simulink model "IEEE34_PQload"  (R2021b)
settings: Solver=ode4  StartTime=0.0  StopTime=5  FixedStep=50e-6  RelTol=1e-3
PreLoadFcn:
  | pGain = 0.05; % Gain of random perturbation (pu)
  | pGainAP = 0.01; % Gain of sinusoidal active power variation (pu)
  | pGainRP = 0.01; % Gain of sinusoidal reactive power variation (pu)
  | pFreqAP = 0.03; % Frequency of sinusoidal active power variation (Hz)
  | pFreqRP = 0.03; % Frequency of sinusoidal reactive power variation (Hz)
  | 
  | init_IEEE34nodetestfeeder;
InitFcn:
  | pGain = 0.05; % Gain of random perturbation (pu)
  | pGainAP = 0.01; % Gain of sinusoidal active power variation (pu)
  | pGainRP = 0.01; % Gain of sinusoidal reactive power variation (pu)
  | pFreqAP = 0.03; % Frequency of sinusoidal active power variation (Hz)
  | pFreqRP = 0.03; % Frequency of sinusoidal reactive power variation (Hz)
  | 
  | init_IEEE34nodetestfeeder;
values from neighbouring files (symbols this model uses):
  fNom = f    (= 60)    [init_IEEE34nodetestfeeder.m]
  loadcoeff = 1.0    (= 1)    [init_IEEE34nodetestfeeder.m]
  Pbase = 500e3    (= 500000)    [init_IEEE34nodetestfeeder.m]
  Ts = 50e-6    (= 5e-05)    [init_IEEE34nodetestfeeder.m]
  vNomMV = VsubL    (= 24900)    [init_IEEE34nodetestfeeder.m]
  VsubL = 24.9e3    (= 24900)    [init_IEEE34nodetestfeeder.m]
undefined symbols (not defined in the file or in its folder): find_system
libraries: spsSeriesRLCBranchLib x330, spsGroundLib x242, LoadLib x88, spsThreePhaseVIMeasurementLib x37, spsMutualInductanceLib x24, spsVoltageMeasurementLib x18, spsCurrentMeasurementLib x12, spsOnDelayLib x12, spsRMSLib x8, spsLinearTransformerLib x6, spsControlledCurrentSourceLib x6, spsControlledVoltageSourceLib x6
(part 2 of 8)

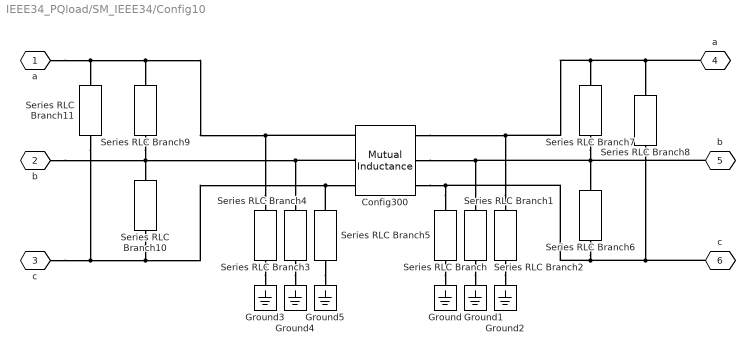
== system IEEE34_PQload/SM_IEEE34/Config10 ==
  Config300 : spsMutualInductanceLib/Mutual Inductance  LConnTagsString=a|b|c  RConnTagsString=A|B|C  TypeOfMutual=Generalized mutual inductance  NumberOfWindings=3  SelfImpedance1=[1.1 1.1e-03]  SelfImpedance2=[ 1.1 1.1e-03]  ThreeWindings=on  SelfImpedance3=[ 1.1 1.1e-03]  MutualImpedance=[1.0 1.0e-03]  InductanceMatrix=[1.3343 0.5779 0.5015 ; 0.5779 1.3569 0.4591; 0.5015 0.4591 1.3471] / (2*fNom*pi) * length/1.6  ResistanceMatrix="[1.3368 0.2101  0.2130 ;  0.2101 1.3238  0.2066;  0.2130 0.2066 1.3294] * length/1.6"  Measurements=None
      settings: SourceProductBaseCode=PS
  Ground{,1..5} (6 alike) : spsGroundLib/Ground  LConnTagsString=a
  Series RLC Branch : spsSeriesRLCBranchLib/Series RLC Branch  LConnTagsString=__new0  RConnTagsString=__new0  BranchType=C  Resistance=1  Inductance=1e-3  SetiL0=off  InitialCurrent=0  Capacitance=1.0417e-8 * length/1.6 / 2  Setx0=off  InitialVoltage=0  Measurements=None
  Series RLC Branch1 : spsSeriesRLCBranchLib/Series RLC Branch  LConnTagsString=__new0  RConnTagsString=__new0  BranchType=C  Resistance=1  Inductance=1e-3  SetiL0=off  InitialCurrent=0  Capacitance=9.3755e-9 * length/1.6 / 2  Setx0=off  InitialVoltage=0  Measurements=None
  Series RLC Branch10 : spsSeriesRLCBranchLib/Series RLC Branch  LConnTagsString=__new0  RConnTagsString=__new0  BranchType=C  Resistance=1  Inductance=1e-3  SetiL0=off  InitialCurrent=0  Capacitance=1.9773e-9 * length/1.6 / 2  Setx0=off  InitialVoltage=0  Measurements=None
  Series RLC Branch11 : spsSeriesRLCBranchLib/Series RLC Branch  LConnTagsString=__new0  RConnTagsString=__new0  BranchType=C  Resistance=1  Inductance=1e-3  SetiL0=off  InitialCurrent=0  Capacitance=3.1650e-9 * length/1.6 / 2  Setx0=off  InitialVoltage=0  Measurements=None
  Series RLC Branch2 : spsSeriesRLCBranchLib/Series RLC Branch  LConnTagsString=__new0  RConnTagsString=__new0  BranchType=C  Resistance=1  Inductance=1e-3  SetiL0=off  InitialCurrent=0  Capacitance=8.9426e-9 * length/1.6 / 2  Setx0=off  InitialVoltage=0  Measurements=None
  Series RLC Branch3 : spsSeriesRLCBranchLib/Series RLC Branch  LConnTagsString=__new0  RConnTagsString=__new0  BranchType=C  Resistance=1  Inductance=1e-3  SetiL0=off  InitialCurrent=0  Capacitance=8.9426e-9 * length/1.6 / 2  Setx0=off  InitialVoltage=0  Measurements=None
  Series RLC Branch4 : spsSeriesRLCBranchLib/Series RLC Branch  LConnTagsString=__new0  RConnTagsString=__new0  BranchType=C  Resistance=1  Inductance=1e-3  SetiL0=off  InitialCurrent=0  Capacitance=9.3755e-9 * length/1.6 / 2  Setx0=off  InitialVoltage=0  Measurements=None
  Series RLC Branch5 : spsSeriesRLCBranchLib/Series RLC Branch  LConnTagsString=__new0  RConnTagsString=__new0  BranchType=C  Resistance=1  Inductance=1e-3  SetiL0=off  InitialCurrent=0  Capacitance=1.0417e-8 * length/1.6 / 2  Setx0=off  InitialVoltage=0  Measurements=None
  Series RLC Branch6 : spsSeriesRLCBranchLib/Series RLC Branch  LConnTagsString=__new0  RConnTagsString=__new0  BranchType=C  Resistance=1  Inductance=1e-3  SetiL0=off  InitialCurrent=0  Capacitance=1.9773e-9 * length/1.6 / 2  Setx0=off  InitialVoltage=0  Measurements=None
  Series RLC Branch7 : spsSeriesRLCBranchLib/Series RLC Branch  LConnTagsString=__new0  RConnTagsString=__new0  BranchType=C  Resistance=1  Inductance=1e-3  SetiL0=off  InitialCurrent=0  Capacitance=4.8743e-9 * length/1.6 / 2  Setx0=off  InitialVoltage=0  Measurements=None
  Series RLC Branch8 : spsSeriesRLCBranchLib/Series RLC Branch  LConnTagsString=__new0  RConnTagsString=__new0  BranchType=C  Resistance=1  Inductance=1e-3  SetiL0=off  InitialCurrent=0  Capacitance=3.1650e-9 * length/1.6 / 2  Setx0=off  InitialVoltage=0  Measurements=None
  Series RLC Branch9 : spsSeriesRLCBranchLib/Series RLC Branch  LConnTagsString=__new0  RConnTagsString=__new0  BranchType=C  Resistance=1  Inductance=1e-3  SetiL0=off  InitialCurrent=0  Capacitance=4.8743e-9 * length/1.6 / 2  Setx0=off  InitialVoltage=0  Measurements=None
  a : PMIOPort  Tag=PMCPort  Side=Left
  b : PMIOPort  Tag=PMCPort  Port=2  Side=Left
  c : PMIOPort  Tag=PMCPort  Port=3  Side=Left
  "a " : PMIOPort  Tag=PMCPort  Port=4  Side=Right
  "b " : PMIOPort  Tag=PMCPort  Port=5  Side=Right
  "c " : PMIOPort  Tag=PMCPort  Port=6  Side=Right
  connections:
  Series RLC Branch3/LConn1 -- Config300/LConn1 -- Series RLC Branch9/LConn1 -- a/RConn1 -- Series RLC Branch11/LConn1
  b/RConn1 -- Series RLC Branch4/LConn1 -- Config300/LConn2 -- Series RLC Branch9/RConn1 -- Series RLC Branch10/LConn1
  Series RLC Branch5/LConn1 -- Config300/LConn3 -- Series RLC Branch10/RConn1 -- c/RConn1 -- Series RLC Branch11/RConn1
  Series RLC Branch2/LConn1 -- Config300/RConn1 -- Series RLC Branch7/LConn1 -- "a "/RConn1 -- Series RLC Branch8/LConn1
  "b "/RConn1 -- Series RLC Branch1/LConn1 -- Config300/RConn2 -- Series RLC Branch6/LConn1 -- Series RLC Branch7/RConn1
  Series RLC Branch/LConn1 -- Config300/RConn3 -- Series RLC Branch6/RConn1 -- "c "/RConn1 -- Series RLC Branch8/RConn1
  Series RLC Branch/RConn1 -- Ground/LConn1
  Series RLC Branch1/RConn1 -- Ground1/LConn1
  Series RLC Branch2/RConn1 -- Ground2/LConn1
  Series RLC Branch3/RConn1 -- Ground3/LConn1
  Series RLC Branch4/RConn1 -- Ground4/LConn1
  Series RLC Branch5/RConn1 -- Ground5/LConn1

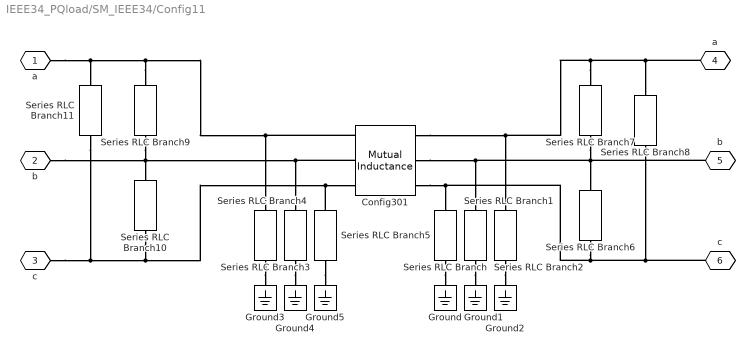
== system IEEE34_PQload/SM_IEEE34/Config11 ==
  Config301 : spsMutualInductanceLib/Mutual Inductance  LConnTagsString=a|b|c  RConnTagsString=A|B|C  TypeOfMutual=Generalized mutual inductance  NumberOfWindings=3  SelfImpedance1=[1.1 1.1e-03]  SelfImpedance2=[ 1.1 1.1e-03]  ThreeWindings=on  SelfImpedance3=[ 1.1 1.1e-03]  MutualImpedance=[1.0 1.0e-03]  InductanceMatrix=[1.4115 0.6442 0.5691 ; 0.6442 1.4281 0.5238; 0.5691 0.5238 1.4209] / (2*fNom*pi) * length/1.6  ResistanceMatrix="[1.9300 0.2327 0.2359 ; 0.2327 1.9157  0.2288;  0.2359 0.2288 1.9219] * length/1.6"  Measurements=None
      settings: SourceProductBaseCode=PS
  Ground{,1..5} (6 alike) : spsGroundLib/Ground  LConnTagsString=a
  Series RLC Branch : spsSeriesRLCBranchLib/Series RLC Branch  LConnTagsString=__new0  RConnTagsString=__new0  BranchType=C  Resistance=1  Inductance=1e-3  SetiL0=off  InitialCurrent=0  Capacitance=1.0123e-8 * length/1.6 / 2  Setx0=off  InitialVoltage=0  Measurements=None
  Series RLC Branch1 : spsSeriesRLCBranchLib/Series RLC Branch  LConnTagsString=__new0  RConnTagsString=__new0  BranchType=C  Resistance=1  Inductance=1e-3  SetiL0=off  InitialCurrent=0  Capacitance=9.1482e-9 * length/1.6 / 2  Setx0=off  InitialVoltage=0  Measurements=None
  Series RLC Branch10 : spsSeriesRLCBranchLib/Series RLC Branch  LConnTagsString=__new0  RConnTagsString=__new0  BranchType=C  Resistance=1  Inductance=1e-3  SetiL0=off  InitialCurrent=0  Capacitance=1.8943e-9 * length/1.6 / 2  Setx0=off  InitialVoltage=0  Measurements=None
  Series RLC Branch11 : spsSeriesRLCBranchLib/Series RLC Branch  LConnTagsString=__new0  RConnTagsString=__new0  BranchType=C  Resistance=1  Inductance=1e-3  SetiL0=off  InitialCurrent=0  Capacitance=2.9927e-9 * length/1.6 / 2  Setx0=off  InitialVoltage=0  Measurements=None
  Series RLC Branch2 : spsSeriesRLCBranchLib/Series RLC Branch  LConnTagsString=__new0  RConnTagsString=__new0  BranchType=C  Resistance=1  Inductance=1e-3  SetiL0=off  InitialCurrent=0  Capacitance=8.7347e-9 * length/1.6 / 2  Setx0=off  InitialVoltage=0  Measurements=None
  Series RLC Branch3 : spsSeriesRLCBranchLib/Series RLC Branch  LConnTagsString=__new0  RConnTagsString=__new0  BranchType=C  Resistance=1  Inductance=1e-3  SetiL0=off  InitialCurrent=0  Capacitance=8.7347e-9 * length/1.6 / 2  Setx0=off  InitialVoltage=0  Measurements=None
  Series RLC Branch4 : spsSeriesRLCBranchLib/Series RLC Branch  LConnTagsString=__new0  RConnTagsString=__new0  BranchType=C  Resistance=1  Inductance=1e-3  SetiL0=off  InitialCurrent=0  Capacitance=9.1482e-9 * length/1.6 / 2  Setx0=off  InitialVoltage=0  Measurements=None
  Series RLC Branch5 : spsSeriesRLCBranchLib/Series RLC Branch  LConnTagsString=__new0  RConnTagsString=__new0  BranchType=C  Resistance=1  Inductance=1e-3  SetiL0=off  InitialCurrent=0  Capacitance=1.0123e-8 * length/1.6 / 2  Setx0=off  InitialVoltage=0  Measurements=None
  Series RLC Branch6 : spsSeriesRLCBranchLib/Series RLC Branch  LConnTagsString=__new0  RConnTagsString=__new0  BranchType=C  Resistance=1  Inductance=1e-3  SetiL0=off  InitialCurrent=0  Capacitance=1.8943e-9 * length/1.6 / 2  Setx0=off  InitialVoltage=0  Measurements=None
  Series RLC Branch7 : spsSeriesRLCBranchLib/Series RLC Branch  LConnTagsString=__new0  RConnTagsString=__new0  BranchType=C  Resistance=1  Inductance=1e-3  SetiL0=off  InitialCurrent=0  Capacitance=4.5722e-9 * length/1.6 / 2  Setx0=off  InitialVoltage=0  Measurements=None
  Series RLC Branch8 : spsSeriesRLCBranchLib/Series RLC Branch  LConnTagsString=__new0  RConnTagsString=__new0  BranchType=C  Resistance=1  Inductance=1e-3  SetiL0=off  InitialCurrent=0  Capacitance=2.9927e-9 * length/1.6 / 2  Setx0=off  InitialVoltage=0  Measurements=None
  Series RLC Branch9 : spsSeriesRLCBranchLib/Series RLC Branch  LConnTagsString=__new0  RConnTagsString=__new0  BranchType=C  Resistance=1  Inductance=1e-3  SetiL0=off  InitialCurrent=0  Capacitance=4.5722e-9 * length/1.6 / 2  Setx0=off  InitialVoltage=0  Measurements=None
  a : PMIOPort  Tag=PMCPort  Side=Left
  b : PMIOPort  Tag=PMCPort  Port=2  Side=Left
  c : PMIOPort  Tag=PMCPort  Port=3  Side=Left
  "a " : PMIOPort  Tag=PMCPort  Port=4  Side=Right
  "b " : PMIOPort  Tag=PMCPort  Port=5  Side=Right
  "c " : PMIOPort  Tag=PMCPort  Port=6  Side=Right
  connections:
  Series RLC Branch9/LConn1 -- a/RConn1 -- Series RLC Branch11/LConn1 -- Config301/LConn1 -- Series RLC Branch3/LConn1
  b/RConn1 -- Series RLC Branch9/RConn1 -- Series RLC Branch10/LConn1 -- Config301/LConn2 -- Series RLC Branch4/LConn1
  Series RLC Branch10/RConn1 -- c/RConn1 -- Series RLC Branch11/RConn1 -- Config301/LConn3 -- Series RLC Branch5/LConn1
  Series RLC Branch7/LConn1 -- "a "/RConn1 -- Series RLC Branch8/LConn1 -- Config301/RConn1 -- Series RLC Branch2/LConn1
  "b "/RConn1 -- Series RLC Branch6/LConn1 -- Series RLC Branch7/RConn1 -- Config301/RConn2 -- Series RLC Branch1/LConn1
  Series RLC Branch6/RConn1 -- "c "/RConn1 -- Series RLC Branch8/RConn1 -- Config301/RConn3 -- Series RLC Branch/LConn1
  Series RLC Branch/RConn1 -- Ground/LConn1
  Series RLC Branch1/RConn1 -- Ground1/LConn1
  Series RLC Branch2/RConn1 -- Ground2/LConn1
  Series RLC Branch3/RConn1 -- Ground3/LConn1
  Series RLC Branch4/RConn1 -- Ground4/LConn1
  Series RLC Branch5/RConn1 -- Ground5/LConn1

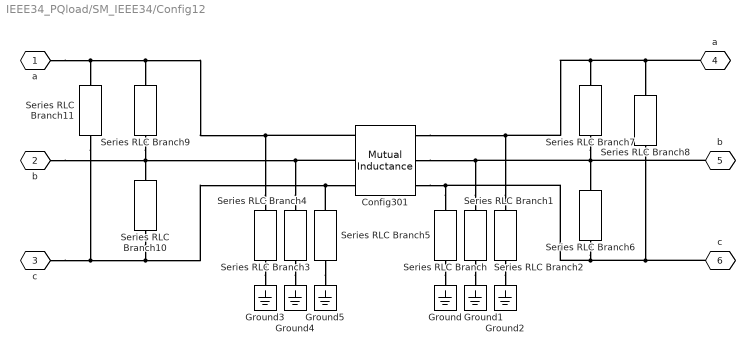
== system IEEE34_PQload/SM_IEEE34/Config12 ==
  Config301 : spsMutualInductanceLib/Mutual Inductance  LConnTagsString=a|b|c  RConnTagsString=A|B|C  TypeOfMutual=Generalized mutual inductance  NumberOfWindings=3  SelfImpedance1=[1.1 1.1e-03]  SelfImpedance2=[ 1.1 1.1e-03]  ThreeWindings=on  SelfImpedance3=[ 1.1 1.1e-03]  MutualImpedance=[1.0 1.0e-03]  InductanceMatrix=[1.4115 0.6442 0.5691 ; 0.6442 1.4281 0.5238; 0.5691 0.5238 1.4209] / (2*fNom*pi) * length/1.6  ResistanceMatrix="[1.9300 0.2327 0.2359 ; 0.2327 1.9157  0.2288;  0.2359 0.2288 1.9219] * length/1.6"  Measurements=None
      settings: SourceProductBaseCode=PS
  Ground{,1..5} (6 alike) : spsGroundLib/Ground  LConnTagsString=a
  Series RLC Branch : spsSeriesRLCBranchLib/Series RLC Branch  LConnTagsString=__new0  RConnTagsString=__new0  BranchType=C  Resistance=1  Inductance=1e-3  SetiL0=off  InitialCurrent=0  Capacitance=1.0123e-8 * length/1.6 / 2  Setx0=off  InitialVoltage=0  Measurements=None
  Series RLC Branch1 : spsSeriesRLCBranchLib/Series RLC Branch  LConnTagsString=__new0  RConnTagsString=__new0  BranchType=C  Resistance=1  Inductance=1e-3  SetiL0=off  InitialCurrent=0  Capacitance=9.1482e-9 * length/1.6 / 2  Setx0=off  InitialVoltage=0  Measurements=None
  Series RLC Branch10 : spsSeriesRLCBranchLib/Series RLC Branch  LConnTagsString=__new0  RConnTagsString=__new0  BranchType=C  Resistance=1  Inductance=1e-3  SetiL0=off  InitialCurrent=0  Capacitance=1.8943e-9 * length/1.6 / 2  Setx0=off  InitialVoltage=0  Measurements=None
  Series RLC Branch11 : spsSeriesRLCBranchLib/Series RLC Branch  LConnTagsString=__new0  RConnTagsString=__new0  BranchType=C  Resistance=1  Inductance=1e-3  SetiL0=off  InitialCurrent=0  Capacitance=2.9927e-9 * length/1.6 / 2  Setx0=off  InitialVoltage=0  Measurements=None
  Series RLC Branch2 : spsSeriesRLCBranchLib/Series RLC Branch  LConnTagsString=__new0  RConnTagsString=__new0  BranchType=C  Resistance=1  Inductance=1e-3  SetiL0=off  InitialCurrent=0  Capacitance=8.7347e-9 * length/1.6 / 2  Setx0=off  InitialVoltage=0  Measurements=None
  Series RLC Branch3 : spsSeriesRLCBranchLib/Series RLC Branch  LConnTagsString=__new0  RConnTagsString=__new0  BranchType=C  Resistance=1  Inductance=1e-3  SetiL0=off  InitialCurrent=0  Capacitance=8.7347e-9 * length/1.6 / 2  Setx0=off  InitialVoltage=0  Measurements=None
  Series RLC Branch4 : spsSeriesRLCBranchLib/Series RLC Branch  LConnTagsString=__new0  RConnTagsString=__new0  BranchType=C  Resistance=1  Inductance=1e-3  SetiL0=off  InitialCurrent=0  Capacitance=9.1482e-9 * length/1.6 / 2  Setx0=off  InitialVoltage=0  Measurements=None
  Series RLC Branch5 : spsSeriesRLCBranchLib/Series RLC Branch  LConnTagsString=__new0  RConnTagsString=__new0  BranchType=C  Resistance=1  Inductance=1e-3  SetiL0=off  InitialCurrent=0  Capacitance=1.0123e-8 * length/1.6 / 2  Setx0=off  InitialVoltage=0  Measurements=None
  Series RLC Branch6 : spsSeriesRLCBranchLib/Series RLC Branch  LConnTagsString=__new0  RConnTagsString=__new0  BranchType=C  Resistance=1  Inductance=1e-3  SetiL0=off  InitialCurrent=0  Capacitance=1.8943e-9 * length/1.6 / 2  Setx0=off  InitialVoltage=0  Measurements=None
  Series RLC Branch7 : spsSeriesRLCBranchLib/Series RLC Branch  LConnTagsString=__new0  RConnTagsString=__new0  BranchType=C  Resistance=1  Inductance=1e-3  SetiL0=off  InitialCurrent=0  Capacitance=4.5722e-9 * length/1.6 / 2  Setx0=off  InitialVoltage=0  Measurements=None
  Series RLC Branch8 : spsSeriesRLCBranchLib/Series RLC Branch  LConnTagsString=__new0  RConnTagsString=__new0  BranchType=C  Resistance=1  Inductance=1e-3  SetiL0=off  InitialCurrent=0  Capacitance=2.9927e-9 * length/1.6 / 2  Setx0=off  InitialVoltage=0  Measurements=None
  Series RLC Branch9 : spsSeriesRLCBranchLib/Series RLC Branch  LConnTagsString=__new0  RConnTagsString=__new0  BranchType=C  Resistance=1  Inductance=1e-3  SetiL0=off  InitialCurrent=0  Capacitance=4.5722e-9 * length/1.6 / 2  Setx0=off  InitialVoltage=0  Measurements=None
  a : PMIOPort  Tag=PMCPort  Side=Left
  b : PMIOPort  Tag=PMCPort  Port=2  Side=Left
  c : PMIOPort  Tag=PMCPort  Port=3  Side=Left
  "a " : PMIOPort  Tag=PMCPort  Port=4  Side=Right
  "b " : PMIOPort  Tag=PMCPort  Port=5  Side=Right
  "c " : PMIOPort  Tag=PMCPort  Port=6  Side=Right
  connections:
  Series RLC Branch5/RConn1 -- Ground5/LConn1
  Series RLC Branch4/RConn1 -- Ground4/LConn1
  Series RLC Branch3/RConn1 -- Ground3/LConn1
  Series RLC Branch2/RConn1 -- Ground2/LConn1
  Series RLC Branch1/RConn1 -- Ground1/LConn1
  Series RLC Branch/RConn1 -- Ground/LConn1
  Series RLC Branch/LConn1 -- Config301/RConn3 -- Series RLC Branch8/RConn1 -- "c "/RConn1 -- Series RLC Branch6/RConn1
  Series RLC Branch1/LConn1 -- Config301/RConn2 -- Series RLC Branch7/RConn1 -- Series RLC Branch6/LConn1 -- "b "/RConn1
  Series RLC Branch2/LConn1 -- Config301/RConn1 -- Series RLC Branch8/LConn1 -- "a "/RConn1 -- Series RLC Branch7/LConn1
  Series RLC Branch5/LConn1 -- Config301/LConn3 -- Series RLC Branch11/RConn1 -- c/RConn1 -- Series RLC Branch10/RConn1
  Series RLC Branch4/LConn1 -- Config301/LConn2 -- Series RLC Branch10/LConn1 -- Series RLC Branch9/RConn1 -- b/RConn1
  Series RLC Branch3/LConn1 -- Config301/LConn1 -- Series RLC Branch11/LConn1 -- a/RConn1 -- Series RLC Branch9/LConn1

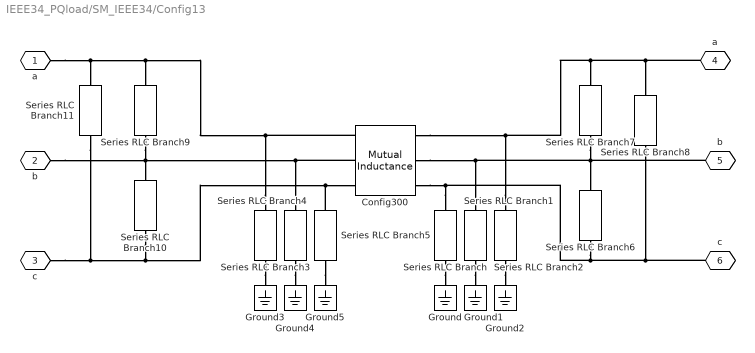
== system IEEE34_PQload/SM_IEEE34/Config13 ==
  Config300 : spsMutualInductanceLib/Mutual Inductance  LConnTagsString=a|b|c  RConnTagsString=A|B|C  TypeOfMutual=Generalized mutual inductance  NumberOfWindings=3  SelfImpedance1=[1.1 1.1e-03]  SelfImpedance2=[ 1.1 1.1e-03]  ThreeWindings=on  SelfImpedance3=[ 1.1 1.1e-03]  MutualImpedance=[1.0 1.0e-03]  InductanceMatrix=[1.3343 0.5779 0.5015 ; 0.5779 1.3569 0.4591; 0.5015 0.4591 1.3471] / (2*fNom*pi) * length/1.6  ResistanceMatrix="[1.3368 0.2101  0.2130 ;  0.2101 1.3238  0.2066;  0.2130 0.2066 1.3294] * length/1.6"  Measurements=None
      settings: SourceProductBaseCode=PS
  Ground{,1..5} (6 alike) : spsGroundLib/Ground  LConnTagsString=a
  Series RLC Branch : spsSeriesRLCBranchLib/Series RLC Branch  LConnTagsString=__new0  RConnTagsString=__new0  BranchType=C  Resistance=1  Inductance=1e-3  SetiL0=off  InitialCurrent=0  Capacitance=(4.8880*1e-6) / (2*fNom*pi) * length/1.6 / 2  Setx0=off  InitialVoltage=0  Measurements=None
  Series RLC Branch1 : spsSeriesRLCBranchLib/Series RLC Branch  LConnTagsString=__new0  RConnTagsString=__new0  BranchType=C  Resistance=1  Inductance=1e-3  SetiL0=off  InitialCurrent=0  Capacitance=(5.0979*1e-6) / (2*fNom*pi) * length/1.6 / 2  Setx0=off  InitialVoltage=0  Measurements=None
  Series RLC Branch10 : spsSeriesRLCBranchLib/Series RLC Branch  LConnTagsString=__new0  RConnTagsString=__new0  BranchType=C  Resistance=1  Inductance=1e-3  SetiL0=off  InitialCurrent=0  Capacitance=(-0.6212*1e-6) / (2*fNom*pi) * length/1.6 / 2  Setx0=off  InitialVoltage=0  Measurements=None
  Series RLC Branch11 : spsSeriesRLCBranchLib/Series RLC Branch  LConnTagsString=__new0  RConnTagsString=__new0  BranchType=C  Resistance=1  Inductance=1e-3  SetiL0=off  InitialCurrent=0  Capacitance=(-0.9943*1e-6) / (2*fNom*pi) * length/1.6 / 2  Setx0=off  InitialVoltage=0  Measurements=None
  Series RLC Branch2 : spsSeriesRLCBranchLib/Series RLC Branch  LConnTagsString=__new0  RConnTagsString=__new0  BranchType=C  Resistance=1  Inductance=1e-3  SetiL0=off  InitialCurrent=0  Capacitance=(5.3350*1e-6) / (2*fNom*pi) * length/1.6 / 2  Setx0=off  InitialVoltage=0  Measurements=None
  Series RLC Branch3 : spsSeriesRLCBranchLib/Series RLC Branch  LConnTagsString=__new0  RConnTagsString=__new0  BranchType=C  Resistance=1  Inductance=1e-3  SetiL0=off  InitialCurrent=0  Capacitance=(5.3350*1e-6) / (2*fNom*pi) * length/1.6 / 2  Setx0=off  InitialVoltage=0  Measurements=None
  Series RLC Branch4 : spsSeriesRLCBranchLib/Series RLC Branch  LConnTagsString=__new0  RConnTagsString=__new0  BranchType=C  Resistance=1  Inductance=1e-3  SetiL0=off  InitialCurrent=0  Capacitance=(5.0979*1e-6) / (2*fNom*pi) * length/1.6 / 2  Setx0=off  InitialVoltage=0  Measurements=None
  Series RLC Branch5 : spsSeriesRLCBranchLib/Series RLC Branch  LConnTagsString=__new0  RConnTagsString=__new0  BranchType=C  Resistance=1  Inductance=1e-3  SetiL0=off  InitialCurrent=0  Capacitance=(4.8880*1e-6) / (2*fNom*pi) * length/1.6 / 2  Setx0=off  InitialVoltage=0  Measurements=None
  Series RLC Branch6 : spsSeriesRLCBranchLib/Series RLC Branch  LConnTagsString=__new0  RConnTagsString=__new0  BranchType=C  Resistance=1  Inductance=1e-3  SetiL0=off  InitialCurrent=0  Capacitance=(-0.6212*1e-6) / (2*fNom*pi) * length/1.6 / 2  Setx0=off  InitialVoltage=0  Measurements=None
  Series RLC Branch7 : spsSeriesRLCBranchLib/Series RLC Branch  LConnTagsString=__new0  RConnTagsString=__new0  BranchType=C  Resistance=1  Inductance=1e-3  SetiL0=off  InitialCurrent=0  Capacitance=(-1.5313*1e-6) / (2*fNom*pi) * length/1.6 / 2  Setx0=off  InitialVoltage=0  Measurements=None
  Series RLC Branch8 : spsSeriesRLCBranchLib/Series RLC Branch  LConnTagsString=__new0  RConnTagsString=__new0  BranchType=C  Resistance=1  Inductance=1e-3  SetiL0=off  InitialCurrent=0  Capacitance=(-0.9943*1e-6) / (2*fNom*pi) * length/1.6 / 2  Setx0=off  InitialVoltage=0  Measurements=None
  Series RLC Branch9 : spsSeriesRLCBranchLib/Series RLC Branch  LConnTagsString=__new0  RConnTagsString=__new0  BranchType=C  Resistance=1  Inductance=1e-3  SetiL0=off  InitialCurrent=0  Capacitance=(-1.5313*1e-6) / (2*fNom*pi) * length/1.6 / 2  Setx0=off  InitialVoltage=0  Measurements=None
  a : PMIOPort  Tag=PMCPort  Side=Left
  b : PMIOPort  Tag=PMCPort  Port=2  Side=Left
  c : PMIOPort  Tag=PMCPort  Port=3  Side=Left
  "a " : PMIOPort  Tag=PMCPort  Port=4  Side=Right
  "b " : PMIOPort  Tag=PMCPort  Port=5  Side=Right
  "c " : PMIOPort  Tag=PMCPort  Port=6  Side=Right
  connections:
  Series RLC Branch3/LConn1 -- Config300/LConn1 -- Series RLC Branch9/LConn1 -- a/RConn1 -- Series RLC Branch11/LConn1
  b/RConn1 -- Series RLC Branch4/LConn1 -- Config300/LConn2 -- Series RLC Branch9/RConn1 -- Series RLC Branch10/LConn1
  Series RLC Branch5/LConn1 -- Config300/LConn3 -- Series RLC Branch10/RConn1 -- c/RConn1 -- Series RLC Branch11/RConn1
  Series RLC Branch2/LConn1 -- Config300/RConn1 -- Series RLC Branch7/LConn1 -- "a "/RConn1 -- Series RLC Branch8/LConn1
  "b "/RConn1 -- Series RLC Branch1/LConn1 -- Config300/RConn2 -- Series RLC Branch6/LConn1 -- Series RLC Branch7/RConn1
  Series RLC Branch/LConn1 -- Config300/RConn3 -- Series RLC Branch6/RConn1 -- "c "/RConn1 -- Series RLC Branch8/RConn1
  Series RLC Branch/RConn1 -- Ground/LConn1
  Series RLC Branch1/RConn1 -- Ground1/LConn1
  Series RLC Branch2/RConn1 -- Ground2/LConn1
  Series RLC Branch3/RConn1 -- Ground3/LConn1
  Series RLC Branch4/RConn1 -- Ground4/LConn1
  Series RLC Branch5/RConn1 -- Ground5/LConn1

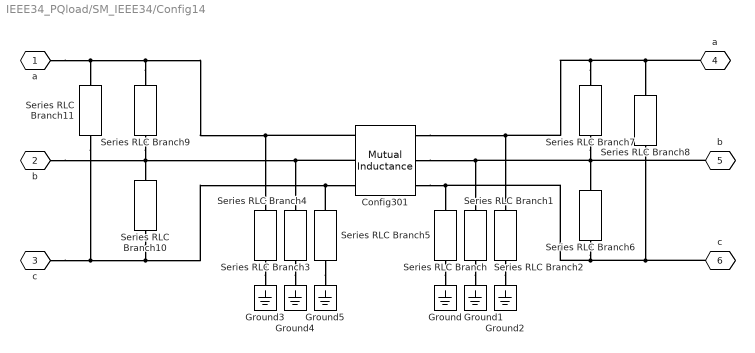
== system IEEE34_PQload/SM_IEEE34/Config14 ==
  Config301 : spsMutualInductanceLib/Mutual Inductance  LConnTagsString=a|b|c  RConnTagsString=A|B|C  TypeOfMutual=Generalized mutual inductance  NumberOfWindings=3  SelfImpedance1=[1.1 1.1e-03]  SelfImpedance2=[ 1.1 1.1e-03]  ThreeWindings=on  SelfImpedance3=[ 1.1 1.1e-03]  MutualImpedance=[1.0 1.0e-03]  InductanceMatrix=[1.4115 0.6442 0.5691 ; 0.6442 1.4281 0.5238; 0.5691 0.5238 1.4209] / (2*fNom*pi) * length/1.6  ResistanceMatrix="[1.9300 0.2327 0.2359 ; 0.2327 1.9157  0.2288;  0.2359 0.2288 1.9219] * length/1.6"  Measurements=None
      settings: SourceProductBaseCode=PS
  Ground{,1..5} (6 alike) : spsGroundLib/Ground  LConnTagsString=a
  Series RLC Branch : spsSeriesRLCBranchLib/Series RLC Branch  LConnTagsString=__new0  RConnTagsString=__new0  BranchType=C  Resistance=1  Inductance=1e-3  SetiL0=off  InitialCurrent=0  Capacitance=1.0123e-8 * length/1.6 / 2  Setx0=off  InitialVoltage=0  Measurements=None
  Series RLC Branch1 : spsSeriesRLCBranchLib/Series RLC Branch  LConnTagsString=__new0  RConnTagsString=__new0  BranchType=C  Resistance=1  Inductance=1e-3  SetiL0=off  InitialCurrent=0  Capacitance=9.1482e-9 * length/1.6 / 2  Setx0=off  InitialVoltage=0  Measurements=None
  Series RLC Branch10 : spsSeriesRLCBranchLib/Series RLC Branch  LConnTagsString=__new0  RConnTagsString=__new0  BranchType=C  Resistance=1  Inductance=1e-3  SetiL0=off  InitialCurrent=0  Capacitance=1.8943e-9 * length/1.6 / 2  Setx0=off  InitialVoltage=0  Measurements=None
  Series RLC Branch11 : spsSeriesRLCBranchLib/Series RLC Branch  LConnTagsString=__new0  RConnTagsString=__new0  BranchType=C  Resistance=1  Inductance=1e-3  SetiL0=off  InitialCurrent=0  Capacitance=2.9927e-9 * length/1.6 / 2  Setx0=off  InitialVoltage=0  Measurements=None
  Series RLC Branch2 : spsSeriesRLCBranchLib/Series RLC Branch  LConnTagsString=__new0  RConnTagsString=__new0  BranchType=C  Resistance=1  Inductance=1e-3  SetiL0=off  InitialCurrent=0  Capacitance=8.7347e-9 * length/1.6 / 2  Setx0=off  InitialVoltage=0  Measurements=None
  Series RLC Branch3 : spsSeriesRLCBranchLib/Series RLC Branch  LConnTagsString=__new0  RConnTagsString=__new0  BranchType=C  Resistance=1  Inductance=1e-3  SetiL0=off  InitialCurrent=0  Capacitance=8.7347e-9 * length/1.6 / 2  Setx0=off  InitialVoltage=0  Measurements=None
  Series RLC Branch4 : spsSeriesRLCBranchLib/Series RLC Branch  LConnTagsString=__new0  RConnTagsString=__new0  BranchType=C  Resistance=1  Inductance=1e-3  SetiL0=off  InitialCurrent=0  Capacitance=9.1482e-9 * length/1.6 / 2  Setx0=off  InitialVoltage=0  Measurements=None
  Series RLC Branch5 : spsSeriesRLCBranchLib/Series RLC Branch  LConnTagsString=__new0  RConnTagsString=__new0  BranchType=C  Resistance=1  Inductance=1e-3  SetiL0=off  InitialCurrent=0  Capacitance=1.0123e-8 * length/1.6 / 2  Setx0=off  InitialVoltage=0  Measurements=None
  Series RLC Branch6 : spsSeriesRLCBranchLib/Series RLC Branch  LConnTagsString=__new0  RConnTagsString=__new0  BranchType=C  Resistance=1  Inductance=1e-3  SetiL0=off  InitialCurrent=0  Capacitance=1.8943e-9 * length/1.6 / 2  Setx0=off  InitialVoltage=0  Measurements=None
  Series RLC Branch7 : spsSeriesRLCBranchLib/Series RLC Branch  LConnTagsString=__new0  RConnTagsString=__new0  BranchType=C  Resistance=1  Inductance=1e-3  SetiL0=off  InitialCurrent=0  Capacitance=4.5722e-9 * length/1.6 / 2  Setx0=off  InitialVoltage=0  Measurements=None
  Series RLC Branch8 : spsSeriesRLCBranchLib/Series RLC Branch  LConnTagsString=__new0  RConnTagsString=__new0  BranchType=C  Resistance=1  Inductance=1e-3  SetiL0=off  InitialCurrent=0  Capacitance=2.9927e-9 * length/1.6 / 2  Setx0=off  InitialVoltage=0  Measurements=None
  Series RLC Branch9 : spsSeriesRLCBranchLib/Series RLC Branch  LConnTagsString=__new0  RConnTagsString=__new0  BranchType=C  Resistance=1  Inductance=1e-3  SetiL0=off  InitialCurrent=0  Capacitance=4.5722e-9 * length/1.6 / 2  Setx0=off  InitialVoltage=0  Measurements=None
  a : PMIOPort  Tag=PMCPort  Side=Left
  b : PMIOPort  Tag=PMCPort  Port=2  Side=Left
  c : PMIOPort  Tag=PMCPort  Port=3  Side=Left
  "a " : PMIOPort  Tag=PMCPort  Port=4  Side=Right
  "b " : PMIOPort  Tag=PMCPort  Port=5  Side=Right
  "c " : PMIOPort  Tag=PMCPort  Port=6  Side=Right
  connections:
  Series RLC Branch9/LConn1 -- a/RConn1 -- Series RLC Branch11/LConn1 -- Config301/LConn1 -- Series RLC Branch3/LConn1
  b/RConn1 -- Series RLC Branch9/RConn1 -- Series RLC Branch10/LConn1 -- Config301/LConn2 -- Series RLC Branch4/LConn1
  Series RLC Branch10/RConn1 -- c/RConn1 -- Series RLC Branch11/RConn1 -- Config301/LConn3 -- Series RLC Branch5/LConn1
  Series RLC Branch7/LConn1 -- "a "/RConn1 -- Series RLC Branch8/LConn1 -- Config301/RConn1 -- Series RLC Branch2/LConn1
  "b "/RConn1 -- Series RLC Branch6/LConn1 -- Series RLC Branch7/RConn1 -- Config301/RConn2 -- Series RLC Branch1/LConn1
  Series RLC Branch6/RConn1 -- "c "/RConn1 -- Series RLC Branch8/RConn1 -- Config301/RConn3 -- Series RLC Branch/LConn1
  Series RLC Branch/RConn1 -- Ground/LConn1
  Series RLC Branch1/RConn1 -- Ground1/LConn1
  Series RLC Branch2/RConn1 -- Ground2/LConn1
  Series RLC Branch3/RConn1 -- Ground3/LConn1
  Series RLC Branch4/RConn1 -- Ground4/LConn1
  Series RLC Branch5/RConn1 -- Ground5/LConn1

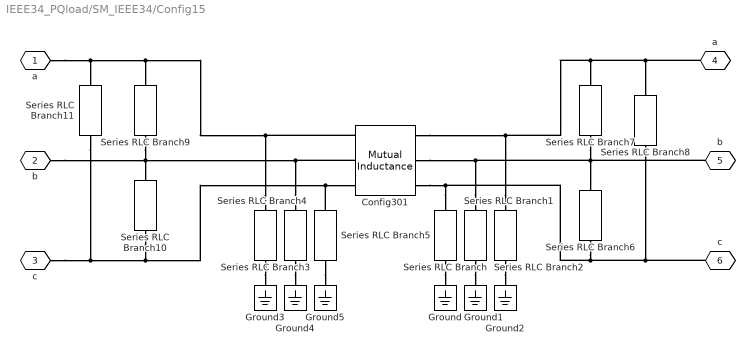
== system IEEE34_PQload/SM_IEEE34/Config15 ==
  Config301 : spsMutualInductanceLib/Mutual Inductance  LConnTagsString=a|b|c  RConnTagsString=A|B|C  TypeOfMutual=Generalized mutual inductance  NumberOfWindings=3  SelfImpedance1=[1.1 1.1e-03]  SelfImpedance2=[ 1.1 1.1e-03]  ThreeWindings=on  SelfImpedance3=[ 1.1 1.1e-03]  MutualImpedance=[1.0 1.0e-03]  InductanceMatrix=[1.4115 0.6442 0.5691 ; 0.6442 1.4281 0.5238; 0.5691 0.5238 1.4209] / (2*fNom*pi) * length/1.6  ResistanceMatrix="[1.9300 0.2327 0.2359 ; 0.2327 1.9157  0.2288;  0.2359 0.2288 1.9219] * length/1.6"  Measurements=None
      settings: SourceProductBaseCode=PS
  Ground{,1..5} (6 alike) : spsGroundLib/Ground  LConnTagsString=a
  Series RLC Branch : spsSeriesRLCBranchLib/Series RLC Branch  LConnTagsString=__new0  RConnTagsString=__new0  BranchType=C  Resistance=1  Inductance=1e-3  SetiL0=off  InitialCurrent=0  Capacitance=1.0123e-8 * length/1.6 / 2  Setx0=off  InitialVoltage=0  Measurements=None
  Series RLC Branch1 : spsSeriesRLCBranchLib/Series RLC Branch  LConnTagsString=__new0  RConnTagsString=__new0  BranchType=C  Resistance=1  Inductance=1e-3  SetiL0=off  InitialCurrent=0  Capacitance=9.1482e-9 * length/1.6 / 2  Setx0=off  InitialVoltage=0  Measurements=None
  Series RLC Branch10 : spsSeriesRLCBranchLib/Series RLC Branch  LConnTagsString=__new0  RConnTagsString=__new0  BranchType=C  Resistance=1  Inductance=1e-3  SetiL0=off  InitialCurrent=0  Capacitance=1.8943e-9 * length/1.6 / 2  Setx0=off  InitialVoltage=0  Measurements=None
  Series RLC Branch11 : spsSeriesRLCBranchLib/Series RLC Branch  LConnTagsString=__new0  RConnTagsString=__new0  BranchType=C  Resistance=1  Inductance=1e-3  SetiL0=off  InitialCurrent=0  Capacitance=2.9927e-9 * length/1.6 / 2  Setx0=off  InitialVoltage=0  Measurements=None
  Series RLC Branch2 : spsSeriesRLCBranchLib/Series RLC Branch  LConnTagsString=__new0  RConnTagsString=__new0  BranchType=C  Resistance=1  Inductance=1e-3  SetiL0=off  InitialCurrent=0  Capacitance=8.7347e-9 * length/1.6 / 2  Setx0=off  InitialVoltage=0  Measurements=None
  Series RLC Branch3 : spsSeriesRLCBranchLib/Series RLC Branch  LConnTagsString=__new0  RConnTagsString=__new0  BranchType=C  Resistance=1  Inductance=1e-3  SetiL0=off  InitialCurrent=0  Capacitance=8.7347e-9 * length/1.6 / 2  Setx0=off  InitialVoltage=0  Measurements=None
  Series RLC Branch4 : spsSeriesRLCBranchLib/Series RLC Branch  LConnTagsString=__new0  RConnTagsString=__new0  BranchType=C  Resistance=1  Inductance=1e-3  SetiL0=off  InitialCurrent=0  Capacitance=9.1482e-9 * length/1.6 / 2  Setx0=off  InitialVoltage=0  Measurements=None
  Series RLC Branch5 : spsSeriesRLCBranchLib/Series RLC Branch  LConnTagsString=__new0  RConnTagsString=__new0  BranchType=C  Resistance=1  Inductance=1e-3  SetiL0=off  InitialCurrent=0  Capacitance=1.0123e-8 * length/1.6 / 2  Setx0=off  InitialVoltage=0  Measurements=None
  Series RLC Branch6 : spsSeriesRLCBranchLib/Series RLC Branch  LConnTagsString=__new0  RConnTagsString=__new0  BranchType=C  Resistance=1  Inductance=1e-3  SetiL0=off  InitialCurrent=0  Capacitance=1.8943e-9 * length/1.6 / 2  Setx0=off  InitialVoltage=0  Measurements=None
  Series RLC Branch7 : spsSeriesRLCBranchLib/Series RLC Branch  LConnTagsString=__new0  RConnTagsString=__new0  BranchType=C  Resistance=1  Inductance=1e-3  SetiL0=off  InitialCurrent=0  Capacitance=4.5722e-9 * length/1.6 / 2  Setx0=off  InitialVoltage=0  Measurements=None
  Series RLC Branch8 : spsSeriesRLCBranchLib/Series RLC Branch  LConnTagsString=__new0  RConnTagsString=__new0  BranchType=C  Resistance=1  Inductance=1e-3  SetiL0=off  InitialCurrent=0  Capacitance=2.9927e-9 * length/1.6 / 2  Setx0=off  InitialVoltage=0  Measurements=None
  Series RLC Branch9 : spsSeriesRLCBranchLib/Series RLC Branch  LConnTagsString=__new0  RConnTagsString=__new0  BranchType=C  Resistance=1  Inductance=1e-3  SetiL0=off  InitialCurrent=0  Capacitance=4.5722e-9 * length/1.6 / 2  Setx0=off  InitialVoltage=0  Measurements=None
  a : PMIOPort  Tag=PMCPort  Side=Left
  b : PMIOPort  Tag=PMCPort  Port=2  Side=Left
  c : PMIOPort  Tag=PMCPort  Port=3  Side=Left
  "a " : PMIOPort  Tag=PMCPort  Port=4  Side=Right
  "b " : PMIOPort  Tag=PMCPort  Port=5  Side=Right
  "c " : PMIOPort  Tag=PMCPort  Port=6  Side=Right
  connections:
  Series RLC Branch5/RConn1 -- Ground5/LConn1
  Series RLC Branch4/RConn1 -- Ground4/LConn1
  Series RLC Branch3/RConn1 -- Ground3/LConn1
  Series RLC Branch2/RConn1 -- Ground2/LConn1
  Series RLC Branch1/RConn1 -- Ground1/LConn1
  Series RLC Branch/RConn1 -- Ground/LConn1
  Series RLC Branch/LConn1 -- Config301/RConn3 -- Series RLC Branch8/RConn1 -- "c "/RConn1 -- Series RLC Branch6/RConn1
  Series RLC Branch1/LConn1 -- Config301/RConn2 -- Series RLC Branch7/RConn1 -- Series RLC Branch6/LConn1 -- "b "/RConn1
  Series RLC Branch2/LConn1 -- Config301/RConn1 -- Series RLC Branch8/LConn1 -- "a "/RConn1 -- Series RLC Branch7/LConn1
  Series RLC Branch5/LConn1 -- Config301/LConn3 -- Series RLC Branch11/RConn1 -- c/RConn1 -- Series RLC Branch10/RConn1
  Series RLC Branch4/LConn1 -- Config301/LConn2 -- Series RLC Branch10/LConn1 -- Series RLC Branch9/RConn1 -- b/RConn1
  Series RLC Branch3/LConn1 -- Config301/LConn1 -- Series RLC Branch11/LConn1 -- a/RConn1 -- Series RLC Branch9/LConn1

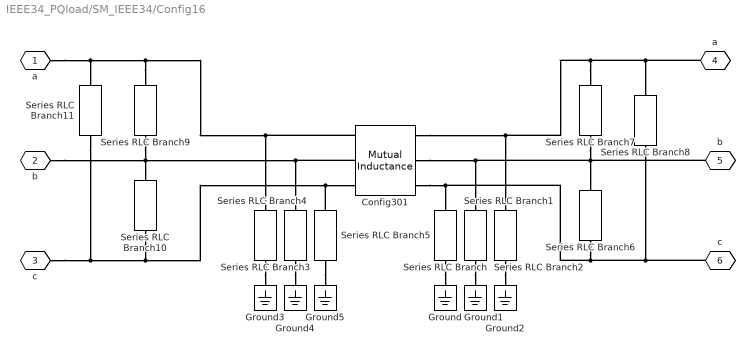
== system IEEE34_PQload/SM_IEEE34/Config16 ==
  Config301 : spsMutualInductanceLib/Mutual Inductance  LConnTagsString=a|b|c  RConnTagsString=A|B|C  TypeOfMutual=Generalized mutual inductance  NumberOfWindings=3  SelfImpedance1=[1.1 1.1e-03]  SelfImpedance2=[ 1.1 1.1e-03]  ThreeWindings=on  SelfImpedance3=[ 1.1 1.1e-03]  MutualImpedance=[1.0 1.0e-03]  InductanceMatrix=[1.4115 0.6442 0.5691 ; 0.6442 1.4281 0.5238; 0.5691 0.5238 1.4209] / (2*fNom*pi) * length/1.6  ResistanceMatrix="[1.9300 0.2327 0.2359 ; 0.2327 1.9157  0.2288;  0.2359 0.2288 1.9219] * length/1.6"  Measurements=None
      settings: SourceProductBaseCode=PS
  Ground{,1..5} (6 alike) : spsGroundLib/Ground  LConnTagsString=a
  Series RLC Branch : spsSeriesRLCBranchLib/Series RLC Branch  LConnTagsString=__new0  RConnTagsString=__new0  BranchType=C  Resistance=1  Inductance=1e-3  SetiL0=off  InitialCurrent=0  Capacitance=1.0123e-8 * length/1.6 / 2  Setx0=off  InitialVoltage=0  Measurements=None
  Series RLC Branch1 : spsSeriesRLCBranchLib/Series RLC Branch  LConnTagsString=__new0  RConnTagsString=__new0  BranchType=C  Resistance=1  Inductance=1e-3  SetiL0=off  InitialCurrent=0  Capacitance=9.1482e-9 * length/1.6 / 2  Setx0=off  InitialVoltage=0  Measurements=None
  Series RLC Branch10 : spsSeriesRLCBranchLib/Series RLC Branch  LConnTagsString=__new0  RConnTagsString=__new0  BranchType=C  Resistance=1  Inductance=1e-3  SetiL0=off  InitialCurrent=0  Capacitance=1.8943e-9 * length/1.6 / 2  Setx0=off  InitialVoltage=0  Measurements=None
  Series RLC Branch11 : spsSeriesRLCBranchLib/Series RLC Branch  LConnTagsString=__new0  RConnTagsString=__new0  BranchType=C  Resistance=1  Inductance=1e-3  SetiL0=off  InitialCurrent=0  Capacitance=2.9927e-9 * length/1.6 / 2  Setx0=off  InitialVoltage=0  Measurements=None
  Series RLC Branch2 : spsSeriesRLCBranchLib/Series RLC Branch  LConnTagsString=__new0  RConnTagsString=__new0  BranchType=C  Resistance=1  Inductance=1e-3  SetiL0=off  InitialCurrent=0  Capacitance=8.7347e-9 * length/1.6 / 2  Setx0=off  InitialVoltage=0  Measurements=None
  Series RLC Branch3 : spsSeriesRLCBranchLib/Series RLC Branch  LConnTagsString=__new0  RConnTagsString=__new0  BranchType=C  Resistance=1  Inductance=1e-3  SetiL0=off  InitialCurrent=0  Capacitance=8.7347e-9 * length/1.6 / 2  Setx0=off  InitialVoltage=0  Measurements=None
  Series RLC Branch4 : spsSeriesRLCBranchLib/Series RLC Branch  LConnTagsString=__new0  RConnTagsString=__new0  BranchType=C  Resistance=1  Inductance=1e-3  SetiL0=off  InitialCurrent=0  Capacitance=9.1482e-9 * length/1.6 / 2  Setx0=off  InitialVoltage=0  Measurements=None
  Series RLC Branch5 : spsSeriesRLCBranchLib/Series RLC Branch  LConnTagsString=__new0  RConnTagsString=__new0  BranchType=C  Resistance=1  Inductance=1e-3  SetiL0=off  InitialCurrent=0  Capacitance=1.0123e-8 * length/1.6 / 2  Setx0=off  InitialVoltage=0  Measurements=None
  Series RLC Branch6 : spsSeriesRLCBranchLib/Series RLC Branch  LConnTagsString=__new0  RConnTagsString=__new0  BranchType=C  Resistance=1  Inductance=1e-3  SetiL0=off  InitialCurrent=0  Capacitance=1.8943e-9 * length/1.6 / 2  Setx0=off  InitialVoltage=0  Measurements=None
  Series RLC Branch7 : spsSeriesRLCBranchLib/Series RLC Branch  LConnTagsString=__new0  RConnTagsString=__new0  BranchType=C  Resistance=1  Inductance=1e-3  SetiL0=off  InitialCurrent=0  Capacitance=4.5722e-9 * length/1.6 / 2  Setx0=off  InitialVoltage=0  Measurements=None
  Series RLC Branch8 : spsSeriesRLCBranchLib/Series RLC Branch  LConnTagsString=__new0  RConnTagsString=__new0  BranchType=C  Resistance=1  Inductance=1e-3  SetiL0=off  InitialCurrent=0  Capacitance=2.9927e-9 * length/1.6 / 2  Setx0=off  InitialVoltage=0  Measurements=None
  Series RLC Branch9 : spsSeriesRLCBranchLib/Series RLC Branch  LConnTagsString=__new0  RConnTagsString=__new0  BranchType=C  Resistance=1  Inductance=1e-3  SetiL0=off  InitialCurrent=0  Capacitance=4.5722e-9 * length/1.6 / 2  Setx0=off  InitialVoltage=0  Measurements=None
  a : PMIOPort  Tag=PMCPort  Side=Left
  b : PMIOPort  Tag=PMCPort  Port=2  Side=Left
  c : PMIOPort  Tag=PMCPort  Port=3  Side=Left
  "a " : PMIOPort  Tag=PMCPort  Port=4  Side=Right
  "b " : PMIOPort  Tag=PMCPort  Port=5  Side=Right
  "c " : PMIOPort  Tag=PMCPort  Port=6  Side=Right
  connections:
  Series RLC Branch9/LConn1 -- a/RConn1 -- Series RLC Branch11/LConn1 -- Config301/LConn1 -- Series RLC Branch3/LConn1
  b/RConn1 -- Series RLC Branch9/RConn1 -- Series RLC Branch10/LConn1 -- Config301/LConn2 -- Series RLC Branch4/LConn1
  Series RLC Branch10/RConn1 -- c/RConn1 -- Series RLC Branch11/RConn1 -- Config301/LConn3 -- Series RLC Branch5/LConn1
  Series RLC Branch7/LConn1 -- "a "/RConn1 -- Series RLC Branch8/LConn1 -- Config301/RConn1 -- Series RLC Branch2/LConn1
  "b "/RConn1 -- Series RLC Branch6/LConn1 -- Series RLC Branch7/RConn1 -- Config301/RConn2 -- Series RLC Branch1/LConn1
  Series RLC Branch6/RConn1 -- "c "/RConn1 -- Series RLC Branch8/RConn1 -- Config301/RConn3 -- Series RLC Branch/LConn1
  Series RLC Branch/RConn1 -- Ground/LConn1
  Series RLC Branch1/RConn1 -- Ground1/LConn1
  Series RLC Branch2/RConn1 -- Ground2/LConn1
  Series RLC Branch3/RConn1 -- Ground3/LConn1
  Series RLC Branch4/RConn1 -- Ground4/LConn1
  Series RLC Branch5/RConn1 -- Ground5/LConn1

== system IEEE34_PQload/SM_IEEE34/Config17 ==
  Config301 : spsMutualInductanceLib/Mutual Inductance  LConnTagsString=a|b|c  RConnTagsString=A|B|C  TypeOfMutual=Generalized mutual inductance  NumberOfWindings=3  SelfImpedance1=[1.1 1.1e-03]  SelfImpedance2=[ 1.1 1.1e-03]  ThreeWindings=on  SelfImpedance3=[ 1.1 1.1e-03]  MutualImpedance=[1.0 1.0e-03]  InductanceMatrix=[1.4115 0.6442 0.5691 ; 0.6442 1.4281 0.5238; 0.5691 0.5238 1.4209] / (2*fNom*pi) * length/1.6  ResistanceMatrix="[1.9300 0.2327 0.2359 ; 0.2327 1.9157  0.2288;  0.2359 0.2288 1.9219] * length/1.6"  Measurements=None
      settings: SourceProductBaseCode=PS
  Ground{,1..5} (6 alike) : spsGroundLib/Ground  LConnTagsString=a
  Series RLC Branch : spsSeriesRLCBranchLib/Series RLC Branch  LConnTagsString=__new0  RConnTagsString=__new0  BranchType=C  Resistance=1  Inductance=1e-3  SetiL0=off  InitialCurrent=0  Capacitance=1.0123e-8 * length/1.6 / 2  Setx0=off  InitialVoltage=0  Measurements=None
  Series RLC Branch1 : spsSeriesRLCBranchLib/Series RLC Branch  LConnTagsString=__new0  RConnTagsString=__new0  BranchType=C  Resistance=1  Inductance=1e-3  SetiL0=off  InitialCurrent=0  Capacitance=9.1482e-9 * length/1.6 / 2  Setx0=off  InitialVoltage=0  Measurements=None
  Series RLC Branch10 : spsSeriesRLCBranchLib/Series RLC Branch  LConnTagsString=__new0  RConnTagsString=__new0  BranchType=C  Resistance=1  Inductance=1e-3  SetiL0=off  InitialCurrent=0  Capacitance=1.8943e-9 * length/1.6 / 2  Setx0=off  InitialVoltage=0  Measurements=None
  Series RLC Branch11 : spsSeriesRLCBranchLib/Series RLC Branch  LConnTagsString=__new0  RConnTagsString=__new0  BranchType=C  Resistance=1  Inductance=1e-3  SetiL0=off  InitialCurrent=0  Capacitance=2.9927e-9 * length/1.6 / 2  Setx0=off  InitialVoltage=0  Measurements=None
  Series RLC Branch2 : spsSeriesRLCBranchLib/Series RLC Branch  LConnTagsString=__new0  RConnTagsString=__new0  BranchType=C  Resistance=1  Inductance=1e-3  SetiL0=off  InitialCurrent=0  Capacitance=8.7347e-9 * length/1.6 / 2  Setx0=off  InitialVoltage=0  Measurements=None
  Series RLC Branch3 : spsSeriesRLCBranchLib/Series RLC Branch  LConnTagsString=__new0  RConnTagsString=__new0  BranchType=C  Resistance=1  Inductance=1e-3  SetiL0=off  InitialCurrent=0  Capacitance=8.7347e-9 * length/1.6 / 2  Setx0=off  InitialVoltage=0  Measurements=None
  Series RLC Branch4 : spsSeriesRLCBranchLib/Series RLC Branch  LConnTagsString=__new0  RConnTagsString=__new0  BranchType=C  Resistance=1  Inductance=1e-3  SetiL0=off  InitialCurrent=0  Capacitance=9.1482e-9 * length/1.6 / 2  Setx0=off  InitialVoltage=0  Measurements=None
  Series RLC Branch5 : spsSeriesRLCBranchLib/Series RLC Branch  LConnTagsString=__new0  RConnTagsString=__new0  BranchType=C  Resistance=1  Inductance=1e-3  SetiL0=off  InitialCurrent=0  Capacitance=1.0123e-8 * length/1.6 / 2  Setx0=off  InitialVoltage=0  Measurements=None
  Series RLC Branch6 : spsSeriesRLCBranchLib/Series RLC Branch  LConnTagsString=__new0  RConnTagsString=__new0  BranchType=C  Resistance=1  Inductance=1e-3  SetiL0=off  InitialCurrent=0  Capacitance=1.8943e-9 * length/1.6 / 2  Setx0=off  InitialVoltage=0  Measurements=None
  Series RLC Branch7 : spsSeriesRLCBranchLib/Series RLC Branch  LConnTagsString=__new0  RConnTagsString=__new0  BranchType=C  Resistance=1  Inductance=1e-3  SetiL0=off  InitialCurrent=0  Capacitance=4.5722e-9 * length/1.6 / 2  Setx0=off  InitialVoltage=0  Measurements=None
  Series RLC Branch8 : spsSeriesRLCBranchLib/Series RLC Branch  LConnTagsString=__new0  RConnTagsString=__new0  BranchType=C  Resistance=1  Inductance=1e-3  SetiL0=off  InitialCurrent=0  Capacitance=2.9927e-9 * length/1.6 / 2  Setx0=off  InitialVoltage=0  Measurements=None
  Series RLC Branch9 : spsSeriesRLCBranchLib/Series RLC Branch  LConnTagsString=__new0  RConnTagsString=__new0  BranchType=C  Resistance=1  Inductance=1e-3  SetiL0=off  InitialCurrent=0  Capacitance=4.5722e-9 * length/1.6 / 2  Setx0=off  InitialVoltage=0  Measurements=None
  a : PMIOPort  Tag=PMCPort  Side=Left
  b : PMIOPort  Tag=PMCPort  Port=2  Side=Left
  c : PMIOPort  Tag=PMCPort  Port=3  Side=Left
  "a " : PMIOPort  Tag=PMCPort  Port=4  Side=Right
  "b " : PMIOPort  Tag=PMCPort  Port=5  Side=Right
  "c " : PMIOPort  Tag=PMCPort  Port=6  Side=Right
  connections:
  Series RLC Branch9/LConn1 -- a/RConn1 -- Series RLC Branch11/LConn1 -- Config301/LConn1 -- Series RLC Branch3/LConn1
  b/RConn1 -- Series RLC Branch9/RConn1 -- Series RLC Branch10/LConn1 -- Config301/LConn2 -- Series RLC Branch4/LConn1
  Series RLC Branch10/RConn1 -- c/RConn1 -- Series RLC Branch11/RConn1 -- Config301/LConn3 -- Series RLC Branch5/LConn1
  Series RLC Branch7/LConn1 -- "a "/RConn1 -- Series RLC Branch8/LConn1 -- Config301/RConn1 -- Series RLC Branch2/LConn1
  "b "/RConn1 -- Series RLC Branch6/LConn1 -- Series RLC Branch7/RConn1 -- Config301/RConn2 -- Series RLC Branch1/LConn1
  Series RLC Branch6/RConn1 -- "c "/RConn1 -- Series RLC Branch8/RConn1 -- Config301/RConn3 -- Series RLC Branch/LConn1
  Series RLC Branch/RConn1 -- Ground/LConn1
  Series RLC Branch1/RConn1 -- Ground1/LConn1
  Series RLC Branch2/RConn1 -- Ground2/LConn1
  Series RLC Branch3/RConn1 -- Ground3/LConn1
  Series RLC Branch4/RConn1 -- Ground4/LConn1
  Series RLC Branch5/RConn1 -- Ground5/LConn1

== system IEEE34_PQload/SM_IEEE34/Config18 ==
  Config301 : spsMutualInductanceLib/Mutual Inductance  LConnTagsString=a|b|c  RConnTagsString=A|B|C  TypeOfMutual=Generalized mutual inductance  NumberOfWindings=3  SelfImpedance1=[1.1 1.1e-03]  SelfImpedance2=[ 1.1 1.1e-03]  ThreeWindings=on  SelfImpedance3=[ 1.1 1.1e-03]  MutualImpedance=[1.0 1.0e-03]  InductanceMatrix=[1.4115 0.6442 0.5691 ; 0.6442 1.4281 0.5238; 0.5691 0.5238 1.4209] / (2*fNom*pi) * length/1.6  ResistanceMatrix="[1.9300 0.2327 0.2359 ; 0.2327 1.9157  0.2288;  0.2359 0.2288 1.9219] * length/1.6"  Measurements=None
      settings: SourceProductBaseCode=PS
  Ground{,1..5} (6 alike) : spsGroundLib/Ground  LConnTagsString=a
  Series RLC Branch : spsSeriesRLCBranchLib/Series RLC Branch  LConnTagsString=__new0  RConnTagsString=__new0  BranchType=C  Resistance=1  Inductance=1e-3  SetiL0=off  InitialCurrent=0  Capacitance=1.0123e-8 * length/1.6 / 2  Setx0=off  InitialVoltage=0  Measurements=None
  Series RLC Branch1 : spsSeriesRLCBranchLib/Series RLC Branch  LConnTagsString=__new0  RConnTagsString=__new0  BranchType=C  Resistance=1  Inductance=1e-3  SetiL0=off  InitialCurrent=0  Capacitance=9.1482e-9 * length/1.6 / 2  Setx0=off  InitialVoltage=0  Measurements=None
  Series RLC Branch10 : spsSeriesRLCBranchLib/Series RLC Branch  LConnTagsString=__new0  RConnTagsString=__new0  BranchType=C  Resistance=1  Inductance=1e-3  SetiL0=off  InitialCurrent=0  Capacitance=1.8943e-9 * length/1.6 / 2  Setx0=off  InitialVoltage=0  Measurements=None
  Series RLC Branch11 : spsSeriesRLCBranchLib/Series RLC Branch  LConnTagsString=__new0  RConnTagsString=__new0  BranchType=C  Resistance=1  Inductance=1e-3  SetiL0=off  InitialCurrent=0  Capacitance=2.9927e-9 * length/1.6 / 2  Setx0=off  InitialVoltage=0  Measurements=None
  Series RLC Branch2 : spsSeriesRLCBranchLib/Series RLC Branch  LConnTagsString=__new0  RConnTagsString=__new0  BranchType=C  Resistance=1  Inductance=1e-3  SetiL0=off  InitialCurrent=0  Capacitance=8.7347e-9 * length/1.6 / 2  Setx0=off  InitialVoltage=0  Measurements=None
  Series RLC Branch3 : spsSeriesRLCBranchLib/Series RLC Branch  LConnTagsString=__new0  RConnTagsString=__new0  BranchType=C  Resistance=1  Inductance=1e-3  SetiL0=off  InitialCurrent=0  Capacitance=8.7347e-9 * length/1.6 / 2  Setx0=off  InitialVoltage=0  Measurements=None
  Series RLC Branch4 : spsSeriesRLCBranchLib/Series RLC Branch  LConnTagsString=__new0  RConnTagsString=__new0  BranchType=C  Resistance=1  Inductance=1e-3  SetiL0=off  InitialCurrent=0  Capacitance=9.1482e-9 * length/1.6 / 2  Setx0=off  InitialVoltage=0  Measurements=None
  Series RLC Branch5 : spsSeriesRLCBranchLib/Series RLC Branch  LConnTagsString=__new0  RConnTagsString=__new0  BranchType=C  Resistance=1  Inductance=1e-3  SetiL0=off  InitialCurrent=0  Capacitance=1.0123e-8 * length/1.6 / 2  Setx0=off  InitialVoltage=0  Measurements=None
  Series RLC Branch6 : spsSeriesRLCBranchLib/Series RLC Branch  LConnTagsString=__new0  RConnTagsString=__new0  BranchType=C  Resistance=1  Inductance=1e-3  SetiL0=off  InitialCurrent=0  Capacitance=1.8943e-9 * length/1.6 / 2  Setx0=off  InitialVoltage=0  Measurements=None
  Series RLC Branch7 : spsSeriesRLCBranchLib/Series RLC Branch  LConnTagsString=__new0  RConnTagsString=__new0  BranchType=C  Resistance=1  Inductance=1e-3  SetiL0=off  InitialCurrent=0  Capacitance=4.5722e-9 * length/1.6 / 2  Setx0=off  InitialVoltage=0  Measurements=None
  Series RLC Branch8 : spsSeriesRLCBranchLib/Series RLC Branch  LConnTagsString=__new0  RConnTagsString=__new0  BranchType=C  Resistance=1  Inductance=1e-3  SetiL0=off  InitialCurrent=0  Capacitance=2.9927e-9 * length/1.6 / 2  Setx0=off  InitialVoltage=0  Measurements=None
  Series RLC Branch9 : spsSeriesRLCBranchLib/Series RLC Branch  LConnTagsString=__new0  RConnTagsString=__new0  BranchType=C  Resistance=1  Inductance=1e-3  SetiL0=off  InitialCurrent=0  Capacitance=4.5722e-9 * length/1.6 / 2  Setx0=off  InitialVoltage=0  Measurements=None
  a : PMIOPort  Tag=PMCPort  Side=Left
  b : PMIOPort  Tag=PMCPort  Port=2  Side=Left
  c : PMIOPort  Tag=PMCPort  Port=3  Side=Left
  "a " : PMIOPort  Tag=PMCPort  Port=4  Side=Right
  "b " : PMIOPort  Tag=PMCPort  Port=5  Side=Right
  "c " : PMIOPort  Tag=PMCPort  Port=6  Side=Right
  connections:
  Series RLC Branch5/RConn1 -- Ground5/LConn1
  Series RLC Branch4/RConn1 -- Ground4/LConn1
  Series RLC Branch3/RConn1 -- Ground3/LConn1
  Series RLC Branch2/RConn1 -- Ground2/LConn1
  Series RLC Branch1/RConn1 -- Ground1/LConn1
  Series RLC Branch/RConn1 -- Ground/LConn1
  Series RLC Branch/LConn1 -- Config301/RConn3 -- Series RLC Branch8/RConn1 -- "c "/RConn1 -- Series RLC Branch6/RConn1
  Series RLC Branch1/LConn1 -- Config301/RConn2 -- Series RLC Branch7/RConn1 -- Series RLC Branch6/LConn1 -- "b "/RConn1
  Series RLC Branch2/LConn1 -- Config301/RConn1 -- Series RLC Branch8/LConn1 -- "a "/RConn1 -- Series RLC Branch7/LConn1
  Series RLC Branch5/LConn1 -- Config301/LConn3 -- Series RLC Branch11/RConn1 -- c/RConn1 -- Series RLC Branch10/RConn1
  Series RLC Branch4/LConn1 -- Config301/LConn2 -- Series RLC Branch10/LConn1 -- Series RLC Branch9/RConn1 -- b/RConn1
  Series RLC Branch3/LConn1 -- Config301/LConn1 -- Series RLC Branch11/LConn1 -- a/RConn1 -- Series RLC Branch9/LConn1
